simulink model "Sim_model_LS"  (R2025a)
settings: Solver=FixedStepAuto  StartTime=0.0  StopTime=40.0  FixedStep=T_sample  RelTol=1e-3
values from neighbouring files (symbols this model uses):
  Ct = 0.65    [loadTCAMParameters.m]
  CTE = 2.4e-4    (= 0.00024)    [loadTCAMParameters.m]
  g = 9.81    [loadTCAMParameters.m]
  m = 400e-3    (= 0.4)    [loadTCAMParameters.m]
  Material = 2    [loadTCAMParameters.m]
  R = 95.0    (= 95)    [loadTCAMParameters.m]
  r0 = 0.4e-3    (= 0.0004)    [loadTCAMParameters.m]
  Ra = 20e6    (= 20000000)    [loadTCAMParameters.m]
  rho = sin(acos(cosbeta_)) / sqrt(m*g/B_)    [loadTCAMParameters.m]
  S = 0.50    (= 0.5)    [loadTCAMParameters.m]
  t1 = 4    [loadTCAMParameters.m]
  T_sample = 0.05    [loadTCAMParameters.m]
  Tamb = 25    [loadTCAMParameters.m]
  V1 = 30    [loadTCAMParameters.m]
settings Model: Creator=thweerakkody  LastModifiedBy=thilinahw
settings RTWCC: GPUComputeCapability=3.5

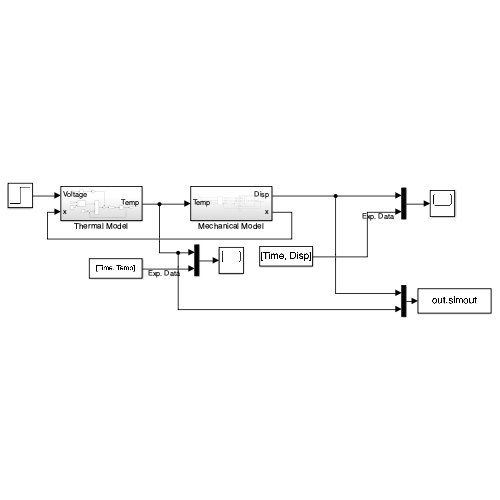
[thumbnail: Simulink's stored preview of the top-level diagram]
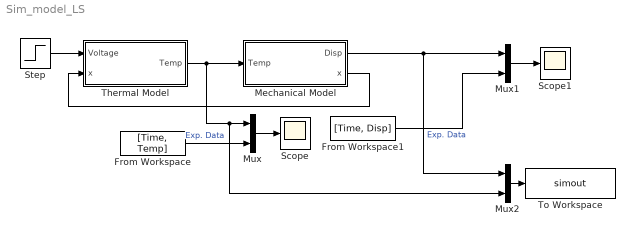
== system Sim_model_LS ==
  From Workspace : FromWorkspace  VariableName=[Time, Temp]
  From Workspace1 : FromWorkspace  VariableName=[Time, Disp]
  Mechanical Model : Subsystem
  Mux : Mux  Inputs=2
  Mux1 : Mux  Inputs=2
  Mux2 : Mux  Inputs=2
  Scope : Scope
      settings: ActiveDisplayYMinimum=18.08288  ActiveDisplayYMaximum=84.30024
  Scope1 : Scope
      settings: ActiveDisplayYMinimum=-0.00118  ActiveDisplayYMaximum=0.01055
  Step : Step  Time=t1  Before=V1  After=0  SampleTime=T_sample
  Thermal Model : Subsystem
  To Workspace : ToWorkspace  VariableName=simout  SaveFormat=Timeseries  SampleTime=-1
  wires:
  Thermal Model/1(Temp) -> Mechanical Model/1(Temp), Mux2/2, Mux/1
  From Workspace/1 -> Mux/2  "Exp. Data"
  Mux/1 -> Scope/1
  Mux1/1 -> Scope1/1
  From Workspace1/1 -> Mux1/2  "Exp. Data"
  Mechanical Model/1(Disp) -> Mux2/1, Mux1/1
  Step/1 -> Thermal Model/1(Voltage)
  Mechanical Model/2(x) -> Thermal Model/2(x)
  Mux2/1 -> To Workspace/1

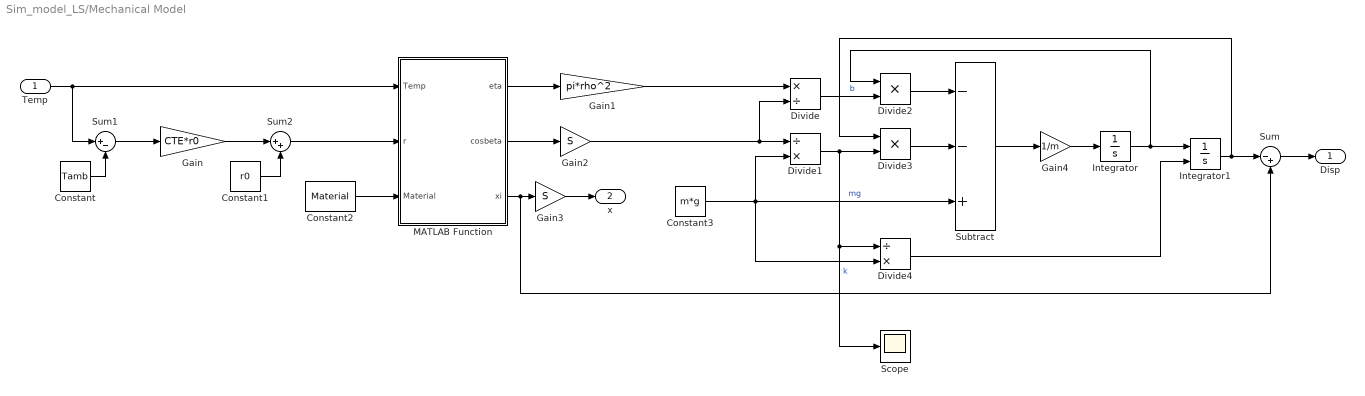
== system Sim_model_LS/Mechanical Model ==
  Temp : Inport
  Constant : Constant  Value=Tamb
  Constant1 : Constant  Value=r0
  Constant2 : Constant  Value=Material
  Constant3 : Constant  Value=m*g
  Divide : Product  Inputs=*/
  Divide1 : Product  Inputs=/*
  Divide2 : Product  Inputs=**
  Divide3 : Product  Inputs=**
  Divide4 : Product  Inputs=/*
  Gain : Gain  Gain=CTE*r0
  Gain1 : Gain  Gain=pi*rho^2
  Gain2 : Gain  Gain=S
  Gain3 : Gain  Gain=S
  Gain4 : Gain  Gain=1/m
  Integrator : Integrator
  Integrator1 : Integrator  InitialConditionSource=external
  MATLAB Function : MATLAB Function  TreatAsAtomicUnit=on
  Scope : Scope
      settings: ActiveDisplayYMinimum=26.48378  ActiveDisplayYMaximum=28.72022
  Subtract : Sum  Inputs=--+
  Sum : Sum  Inputs=|-+
  Sum1 : Sum  Inputs=|+-
  Sum2 : Sum  Inputs=|++
  Disp : Outport
  x : Outport  Port=2
  wires:
  Constant2/1 -> MATLAB Function/3(Material)
  MATLAB Function/1(eta) -> Gain1/1
  MATLAB Function/2(cosbeta) -> Gain2/1
  Sum/1 -> Disp/1
  Temp/1 -> MATLAB Function/1(Temp), Sum1/1
  Constant/1 -> Sum1/2
  Sum1/1 -> Gain/1
  Gain/1 -> Sum2/1
  Constant1/1 -> Sum2/2
  Sum2/1 -> MATLAB Function/2(r)
  Gain1/1 -> Divide/1
  Gain2/1 -> Divide/2, Divide1/1
  MATLAB Function/3(xi) -> Sum/2, Gain3/1
  Gain3/1 -> x/1
  Constant3/1 -> Divide4/2, Divide1/2, Subtract/3  "mg"
  Divide/1 -> Divide2/2  "b"
  Divide1/1 -> Scope/1, Divide4/1, Divide3/2  "k"
  Divide2/1 -> Subtract/1
  Divide3/1 -> Subtract/2
  Subtract/1 -> Gain4/1
  Gain4/1 -> Integrator/1
  Integrator/1 -> Divide2/1, Integrator1/1
  Divide4/1 -> Integrator1/2
  Integrator1/1 -> Divide3/1, Sum/1

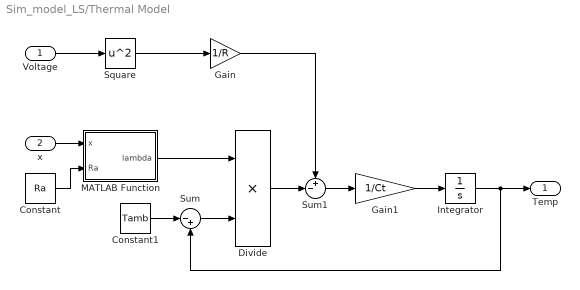
== system Sim_model_LS/Thermal Model ==
  Voltage : Inport
  x : Inport  Port=2
  Constant : Constant  Value=Ra
  Constant1 : Constant  Value=Tamb
  Divide : Product  Inputs=**
  Gain : Gain  Gain=1/R
  Gain1 : Gain  Gain=1/Ct
  Integrator : Integrator  InitialCondition=Tamb
  MATLAB Function : MATLAB Function  TreatAsAtomicUnit=on
  Square : Math  Operator=square
  Sum : Sum  Inputs=|-+
  Sum1 : Sum  Inputs=+-|
  Temp : Outport
  wires:
  x/1 -> MATLAB Function/1(x)
  Voltage/1 -> Square/1
  Square/1 -> Gain/1
  Constant/1 -> MATLAB Function/2(Ra)
  Sum/1 -> Divide/2
  MATLAB Function/1(lambda) -> Divide/1
  Constant1/1 -> Sum/1
  Gain/1 -> Sum1/1
  Divide/1 -> Sum1/2
  Sum1/1 -> Gain1/1
  Gain1/1 -> Integrator/1
  Integrator/1 -> Sum/2, Temp/1

== matlab function Sim_model_LS/Mechanical Model/MATLAB Function ==
  settings: updateMethod=DISCRETE
  data: Temp input; r input; eta output; Material input; cosbeta output; xi output
function [eta, cosbeta, xi] = fcn(Temp, r, Material)
persistent m n S r0 alpha_deg vf;
if Material==1
    m = 50e-3;      % Fabrication mass [kg]
    n = 120;        % number of coiled turns
    S = 0.25;       % Initial fiber length [m]
    r0 = 0.29e-3;   % Initial fiber radius [m]
    alpha_deg = 5;  % Twisting angle [deg]
    vf  = 0.975;    % Volume fraction
else
    m = 400e-3;     % Fabrication mass [kg]
    n = 240;        % number of coiled turns
    S = 0.5;        % Initial fiber length [m]
    r0 = 0.4e-3;    % Initial fiber radius [m]
    alpha_deg = 5;  % Twisting angle [deg]
    vf  = 0.99;     % Volume fraction
end

alpha = deg2rad(alpha_deg);% Twisting angle [rad]
g = 9.81;                  % gravity [m/s^2]
q = 2*pi*n/S;
Em  = 3e6;
nim = 0.5;
Gm  = Em/(2*(1+nim));
Ef1 = 230*10^9;             %STATIC:page 12
Ef2 = 16*10^9;
Gf12= 14*10^9;
nif12 = 0.2;
nif23 = 0.31;

%% volumetric fractions
vm = 1-vf;                    %STATIC:eq (A2)

%compliance matrix impregnated STRAIGHT FIBER (Ort Transv Isotr)
E11 = vf*Ef1+vm*Em;                         %STATIC:eq (A2)
E22 = Em*((1-(vf)^0.5)+(vf)^0.5/(1-(vf)^0.5*(1-(Em/Ef2))));%STATIC:eq (A5)
ni12= vf*nif12+vm*nim;
ni21= ni12*E22/E11;                         %STATIC:eq (A3)
ni23= vf*nif23+vm*nim;                      %STATIC:eq (A4)
G12 = Gm*((1-(vf)^0.5)+(vf)^0.5/(1-(vf)^0.5*(1-(Gm/Gf12))));%STATIC:eq (A6)
S11 = 1/E11;                                %STATIC:eq (A8)
S22 = 1/E22;
S12 =-ni21/E22;
S23 =-ni23/E22;
S44 = 2*(1+ni23)/E22;
S66 = 1/G12;

%% Compliance matrix IMPREGNATED TWISTED FIBER
c  = cos(alpha);
s  = sin(alpha);
S11a = S11*c^4+S22*s^4+(2*S12+S66)*c^2*s^2;%STATIC:eq (A7)
S12a = 0.5*((S11+S22-S66)*c^2*s^2+S12*(c^4+s^4+c^2)+S23*s^2);
S22a = 0.125*(3*S11*s^4+(2*S12+S66)*(1+3*c^2)*s^2+3*S22*(1+c^4)+(2*S23+S44)*c^2);
S23a = 0.125*(S11*s^4+2*S12*c^2*s^2+S22*(1+c^4)-S44*c^2-S66*s^4+6*(S12*s^2+S23*c^2));
S44a = 0.5*((S11-2*S12)*s^4+S22*(1+c^4)+(S44-2*S23)*c^2+S66*s^2*(1+c^2));
S55a = 2*(S11-2*S12+S22)*c^2*s^2+0.5*(S66*(c^2+(cos(2*alpha))^2)+S44*s^2);
S66a = S55a;

%% Compliance matrix IMPREGNATED TWISTED YARN
ct2= (cot(alpha))^2;                       
I1 = 0.5*(ct2)*(1-c^2+s^2);
I2 = 2*ct2*(0.5/(c^2)+2*log(c)-0.5*c^2);
I3 = 2*ct2*log(sec(alpha));
I4 = 2*ct2*((c^2)/2-log(c)-0.5);
I5 = 2*ct2*(log(c)+0.5/(c^2)-0.5);
I6 = 2*ct2*(0.5*s^2/(c^2));
S11y = S11a*I1+S22a*I2+(2*S12a+S66a)*I4;
S44y=0.5*((S11a-2*S12a)*I2+S22a*(I6+I1)+(S44a-2*S23a)*I3+S66a*(I5+I4));
Ex=1/S11y;                                  
Gyz=1/S44y;                                 

%% 
B_ = Ex*pi*r0^4/4;                               
C_ = Gyz*pi*r0^4/2;                             
cosbeta_ = 1-(1/(B_-C_))*(q*B_*C_/sqrt(B_*m*g)-2*C_);   
xi = S*cosbeta_ ;  

%%
B = Ex*pi/4*r^4;
C = Gyz*pi/2*r^4;
cosbeta = 1-(1/(B-C))*(q*B*C/sqrt(B*m*g)-2*C);
                      

%% Viscosity calculation 
knu = 5.1/1030;
eta = (1239-9.19e-1*(Temp+273.15))*knu*100; % Viscosity [Pa.s]

== matlab function Sim_model_LS/Thermal Model/MATLAB Function ==
  data: x input; lambda output; Ra input
function lambda= fcn(x, Ra)
Pr = 0.71;          % Prandtl number
k_heat = 28e-3;     % Thermal conductivity of the TCAM
rho = 0.0082;       % Initial radius of the coil
Nu = ((((Ra^(1/6))*0.387)/(((0.559/Pr)^(9/16)+1)^(8/27)))+0.6)^2;
h  = k_heat*Nu/(x);% Convection heat transfer coefficient
As = 2*pi*rho*x;   % Effective cross-section area of the TCAM
lambda = h*As;
